simulink model "rlsdemo"  (Simulink 5.0)
settings: Solver=FixedStepDiscrete  StartTime=0  StopTime=inf  RelTol=1e-3  AbsTol=1e-6
libraries: dspsnks4 x2, simulink x2, dspsrcs4 x2, dsparch4 x1, dspadpt3 x1
Description:
  | RLS adaptive noise cancellation
settings Model: CovMetricSettings=d  Creator=don  LastModifiedBy=mkhan  ExtModeTrigMode=oneshot  ExtModeArmWhenConnect=off  ExtModeAutoUpdateStatusClock=off  SaveTime=off  SaveOutput=off  LimitDataPoints=off  IntegerOverflowMsg=none  ZeroCrossControl=UseLocalSettings  ProdHWWordLengths=8,32,16,32  TargetHWChar=2  TargetHWWordLengths=8,16,32,32  RTWMathFcnLibMatFile=iso_c_tmw.mat  RTWOptions="-aEnforceIntegerDowncast=1 -aFoldNonRolledExpr=1 -aInlineInvariantSignals=0 -aInlineParameters=0 -aLocalBlockOutputs=1 -aRollThreshold=5 -aRTWVerbose=1 -aForceParamTrailComments=0 -aGenerateComments=1 -aIgnoreCustomStorageClasses=1 -aIncHierarchyInIds=0 -aMaxRTWIdLen=31 -aShowEliminatedStatements=0 -aReadOnly=0 -aTargetFcnLib=\"iso_c_tmw.mat\" -aIncDataTypeInIds=0 -aPrefixModelToSubsysFcnNames=1 -aInlinedPrmAccess=\"Literals\" -aGenerateFullHeader=1 -aIsPILTarget=0 -aGenerateReport=0 -aLogVarNameModifier=\"rt_\" -aExtMode=0 -aExtModeStaticAlloc=0 -aExtModeTesting=0 -aExtModeStaticAllocSize=1000000 -aExtModeTransport=0  -aExtModeTransport=\"tcpip\""

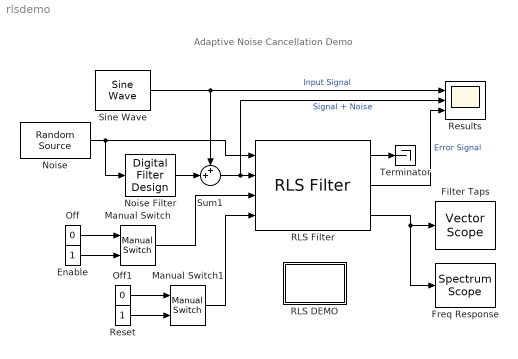
== system rlsdemo ==
  note: Adaptive Noise Cancellation Demo
  Enable : Constant  ShowAdditionalParam=on  OutDataTypeMode=boolean
  Filter Taps : dspsnks4/Vector Scope  ScopeProperties=off  Domain=User-defined  HorizSpan=1  DisplayProperties=off  AxisGrid=on  Memory=off  FrameNumber=on  AxisLegend=off  AxisZoom=on  OpenScopeAtSimStart=on  OpenScopeImmediately=off  FigPos=[31 183 329 270]  AxisProperties=on  XUnits=Hertz  XRange=[0...Fs/2]  InheritXIncr=on  XIncr=1  XLabel=Samples  YUnits=dB  YLabel=Filter Coefficients  LineProperties=off  LineDisables=on  LineStyles=:  LineMarkers=.  LineColors=[0 0 1]
      settings: YMin=-0.2  YMax=0.6
  Freq Response : dspsnks4/Spectrum Scope  ScopeProperties=off  Domain=Frequency  HorizSpan=1  UseBuffer=off  BufferSize=128  Overlap=64  inpFftLenInherit=on  FFTlength=256  numAvg=2  DisplayProperties=off  AxisGrid=on  Memory=off  FrameNumber=on  AxisLegend=off  AxisZoom=on  OpenScopeAtSimStart=on  OpenScopeImmediately=off  FigPos=[369 182 378 270]  AxisProperties=on  XUnits=Hertz  XRange=[0...Fs/2]  InheritXIncr=on  XIncr=1  XLabel=Samples  YUnits=dB  YLabel=Magnitude, dB  LineProperties=off  LineDisables=on  LineStyles=-  LineColors=[0 0 1]
      settings: YMin=-60  YMax=0
  Manual Switch : simulink/Signal Routing/Manual Switch  sw=0  action=0
  Manual Switch1 : simulink/Signal Routing/Manual Switch  sw=1  action=0
  Noise : dspsrcs4/Random Source  SrcType=Gaussian  NormMethod=Ziggurat  CltLength=12  Min=0  Max=1  Mean=0  Var=1  RepMode=Specify seed  Seed=[23341]  Inherit=off  SampMode=Discrete  SampTime=1  SampFrame=1  DataType=Double  OutComplex=Real
  Noise Filter : dsparch4/Digital Filter Design
  Off : Constant  Value=0  ShowAdditionalParam=on  OutDataTypeMode=boolean
  Off1 : Constant  Value=0  ShowAdditionalParam=on  OutDataTypeMode=boolean
  RLS DEMO : Subsystem
      mask Display: disp('Info')
  RLS Filter : dspadpt3/RLS Filter  L=32  lambdaflag=Dialog  lambda=1.0  addnparflag=on  ic=0  delta=0.1  Adapt=on  resetflag=Either edge  weights=on
  Reset : Constant  ShowAdditionalParam=on  OutDataTypeMode=boolean
  Results : Scope  NumInputPorts=3
      settings: TimeRange=128  YMin=-2~-2~-2  YMax=2~2~2  DataFormat=Array
  Sine Wave : dspsrcs4/Sine Wave  Amplitude=1  Frequency=0.055  Phase=0  SampleMode=Discrete  OutComplex=Real  CompMethod=Trigonometric fcn  TableSize=Speed  SampleTime=1  SamplesPerFrame=1  dataType=double  wordLen=16  udDataType=sfix(16)  fracBitsMode=User-defined  numFracBits=14  ResetState=Restart at time zero
  Sum1 : Sum  Inputs=++|  SaturateOnIntegerOverflow=on  InputSameDT=on
  Terminator : Terminator
  wires:
  Sine Wave/1 -> Results/1, Sum1/1  "Input Signal"
  Noise Filter/1 -> Sum1/2
  Noise/1 -> RLS Filter/1, Noise Filter/1
  Sum1/1 -> Results/2, RLS Filter/2  "Signal + Noise"
  RLS Filter/2 -> Results/3  "Error Signal"
  RLS Filter/1 -> Terminator/1
  RLS Filter/3 -> Freq Response/1, Filter Taps/1
  Off/1 -> Manual Switch/1
  Enable/1 -> Manual Switch/2
  Off1/1 -> Manual Switch1/1
  Reset/1 -> Manual Switch1/2
  Manual Switch/1 -> RLS Filter/3
  Manual Switch1/1 -> RLS Filter/4

== system rlsdemo/RLS DEMO ==
  note: Adaptive Noise Cancellation using the Recursive
      | Least Squares Algorithm.
      |
      | The RLS adaptive filter uses the reference signal (on
      | the "Input" port) and the "Desired" signal to automatically match the filter
      | response in the block labeled "Noise filter". As it converges to
      | the correct filter, the filtered noise should be
      | completely subtracted from the "Signal+Noise" signal
      | and the "Error Signal" should contain only
      | the original signal.
      |
      | For details, see "Adaptive Filter Theory", 3rd Ed. by
      | S. Haykin, Prentice-Hall 1996.
